simulink subsystem "parallel_to_serial"  (R2022b)
settings: Solver=VariableStepAuto  StartTime=0.0  StopTime=10.0  RelTol=1e-3
settings Model: Creator=Ali-Laptop  LastModifiedBy=Ali-Laptop

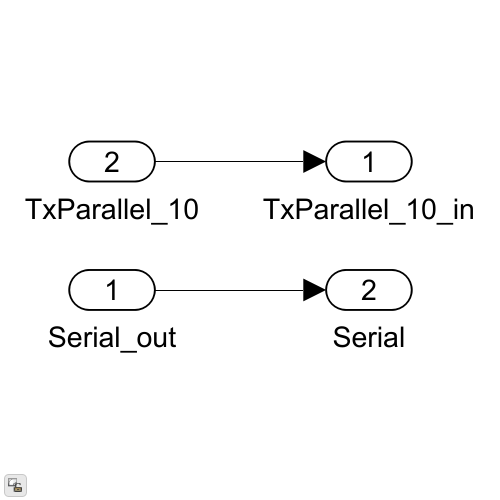
[thumbnail: Simulink's stored preview of the top-level diagram]
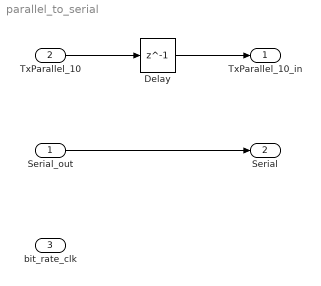
== system parallel_to_serial ==
  Serial_out : Inport
  TxParallel_10 : Inport  Port=2
  bit_rate_clk : Inport  Port=3
  Delay : Delay  DelayLength=1
  TxParallel_10_in : Outport
  Serial : Outport  Port=2
  wires:
  TxParallel_10/1 -> Delay/1
  Serial_out/1 -> Serial/1
  Delay/1 -> TxParallel_10_in/1
